simulink model "LGS_allFaultsDeselected"  (R2019b)
settings: Solver=FixedStepDiscrete  StartTime=0.0  StopTime=45.0  FixedStep=0.1  RelTol=1e-3
model workspace (MAT data in the model file):
  fipData : object (value not decoded)
  fipName : object (value not decoded)
  stepSize = 0.1
libraries: LibFaultInjectionControls x190, commrandsrc3 x70, simulink x3, LibFailureCondition x1
(part 7 of 41)

== system LGS_allFaultsDeselected/Digital Part/Computing module2/GenericMonitoring3 ==
  In1 : Inport
  AND : Logic  Inputs=3  IconShape=distinctive  AllPortsSameDT=off  OutDataTypeStr=boolean
  Bus Selector : BusSelector  OutputSignals=signal1,signal2,signal3
  GenericMonitoring2 : Stateflow chart  TreatAsAtomicUnit=on
  Logical Operator1 : Logic  Operator=XOR  AllPortsSameDT=off  OutDataTypeStr=boolean
  Logical Operator2 : Logic  Operator=XOR  AllPortsSameDT=off  OutDataTypeStr=boolean
  Logical Operator3 : Logic  Operator=NOT  AllPortsSameDT=off  OutDataTypeStr=boolean
  Logical Operator4 : Logic  Operator=NOT  AllPortsSameDT=off  OutDataTypeStr=boolean
  Switch : Switch  Criteria=u2 > Threshold
  Switch1 : Switch  Criteria=u2 > Threshold
  Switch2 : Switch  Criteria=u2 > Threshold
  Signal : Outport  OutDataTypeStr=boolean
  Anomaly : Outport  Port=2  OutDataTypeStr=boolean
  wires:
  Bus Selector/1 -> GenericMonitoring2/1(Channel1), Logical Operator1/1, Switch1/1, Switch/1, AND/1  "<signal1>"
  Bus Selector/2 -> AND/2, GenericMonitoring2/2(Channel2), Logical Operator1/2, Logical Operator2/1, Switch2/1  "<signal2>"
  Bus Selector/3 -> AND/3, GenericMonitoring2/3(Channel3), Logical Operator2/2, Switch2/3  "<signal3>"
  In1/1 -> Bus Selector/1
  AND/1 -> Switch/2
  GenericMonitoring2/1(anomaly) -> Anomaly/1
  Switch/1 -> Signal/1
  Logical Operator4/1 -> Switch1/2
  Logical Operator2/1 -> Logical Operator3/1
  Switch2/1 -> Switch1/3
  Switch1/1 -> Switch/3
  Logical Operator3/1 -> Switch2/2
  Logical Operator1/1 -> Logical Operator4/1

== system LGS_allFaultsDeselected/Digital Part/Computing module2/GenericMonitoring4 ==
  In1 : Inport
  AND : Logic  Inputs=3  IconShape=distinctive  AllPortsSameDT=off  OutDataTypeStr=boolean
  Bus Selector : BusSelector  OutputSignals=signal1,signal2,signal3
  GenericMonitoring2 : Stateflow chart  TreatAsAtomicUnit=on
  Logical Operator1 : Logic  Operator=XOR  AllPortsSameDT=off  OutDataTypeStr=boolean
  Logical Operator2 : Logic  Operator=XOR  AllPortsSameDT=off  OutDataTypeStr=boolean
  Logical Operator3 : Logic  Operator=NOT  AllPortsSameDT=off  OutDataTypeStr=boolean
  Logical Operator4 : Logic  Operator=NOT  AllPortsSameDT=off  OutDataTypeStr=boolean
  Switch : Switch  Criteria=u2 > Threshold
  Switch1 : Switch  Criteria=u2 > Threshold
  Switch2 : Switch  Criteria=u2 > Threshold
  Signal : Outport  OutDataTypeStr=boolean
  Anomaly : Outport  Port=2  OutDataTypeStr=boolean
  wires:
  Bus Selector/1 -> GenericMonitoring2/1(Channel1), Logical Operator1/1, Switch1/1, Switch/1, AND/1  "<signal1>"
  Bus Selector/2 -> AND/2, GenericMonitoring2/2(Channel2), Logical Operator1/2, Logical Operator2/1, Switch2/1  "<signal2>"
  Bus Selector/3 -> AND/3, GenericMonitoring2/3(Channel3), Logical Operator2/2, Switch2/3  "<signal3>"
  In1/1 -> Bus Selector/1
  AND/1 -> Switch/2
  GenericMonitoring2/1(anomaly) -> Anomaly/1
  Switch/1 -> Signal/1
  Logical Operator4/1 -> Switch1/2
  Logical Operator2/1 -> Logical Operator3/1
  Switch2/1 -> Switch1/3
  Switch1/1 -> Switch/3
  Logical Operator3/1 -> Switch2/2
  Logical Operator1/1 -> Logical Operator4/1

== system LGS_allFaultsDeselected/Digital Part/Computing module2/GenericMonitoring5 ==
  In1 : Inport
  AND : Logic  Inputs=3  IconShape=distinctive  AllPortsSameDT=off  OutDataTypeStr=boolean
  Bus Selector : BusSelector  OutputSignals=signal1,signal2,signal3
  GenericMonitoring2 : Stateflow chart  TreatAsAtomicUnit=on
  Logical Operator1 : Logic  Operator=XOR  AllPortsSameDT=off  OutDataTypeStr=boolean
  Logical Operator2 : Logic  Operator=XOR  AllPortsSameDT=off  OutDataTypeStr=boolean
  Logical Operator3 : Logic  Operator=NOT  AllPortsSameDT=off  OutDataTypeStr=boolean
  Logical Operator4 : Logic  Operator=NOT  AllPortsSameDT=off  OutDataTypeStr=boolean
  Switch : Switch  Criteria=u2 > Threshold
  Switch1 : Switch  Criteria=u2 > Threshold
  Switch2 : Switch  Criteria=u2 > Threshold
  Signal : Outport  OutDataTypeStr=boolean
  Anomaly : Outport  Port=2  OutDataTypeStr=boolean
  wires:
  Bus Selector/1 -> GenericMonitoring2/1(Channel1), Logical Operator1/1, Switch1/1, Switch/1, AND/1  "<signal1>"
  Bus Selector/2 -> AND/2, GenericMonitoring2/2(Channel2), Logical Operator1/2, Logical Operator2/1, Switch2/1  "<signal2>"
  Bus Selector/3 -> AND/3, GenericMonitoring2/3(Channel3), Logical Operator2/2, Switch2/3  "<signal3>"
  In1/1 -> Bus Selector/1
  AND/1 -> Switch/2
  GenericMonitoring2/1(anomaly) -> Anomaly/1
  Switch/1 -> Signal/1
  Logical Operator4/1 -> Switch1/2
  Logical Operator2/1 -> Logical Operator3/1
  Switch2/1 -> Switch1/3
  Switch1/1 -> Switch/3
  Logical Operator3/1 -> Switch2/2
  Logical Operator1/1 -> Logical Operator4/1

== system LGS_allFaultsDeselected/Digital Part/Computing module2/GenericMonitoring6 ==
  In1 : Inport
  AND : Logic  Inputs=3  IconShape=distinctive  AllPortsSameDT=off  OutDataTypeStr=boolean
  Bus Selector : BusSelector  OutputSignals=signal1,signal2,signal3
  GenericMonitoring2 : Stateflow chart  TreatAsAtomicUnit=on
  Logical Operator1 : Logic  Operator=XOR  AllPortsSameDT=off  OutDataTypeStr=boolean
  Logical Operator2 : Logic  Operator=XOR  AllPortsSameDT=off  OutDataTypeStr=boolean
  Logical Operator3 : Logic  Operator=NOT  AllPortsSameDT=off  OutDataTypeStr=boolean
  Logical Operator4 : Logic  Operator=NOT  AllPortsSameDT=off  OutDataTypeStr=boolean
  Switch : Switch  Criteria=u2 > Threshold
  Switch1 : Switch  Criteria=u2 > Threshold
  Switch2 : Switch  Criteria=u2 > Threshold
  Signal : Outport  OutDataTypeStr=boolean
  Anomaly : Outport  Port=2  OutDataTypeStr=boolean
  wires:
  Bus Selector/1 -> GenericMonitoring2/1(Channel1), Logical Operator1/1, Switch1/1, Switch/1, AND/1  "<signal1>"
  Bus Selector/2 -> AND/2, GenericMonitoring2/2(Channel2), Logical Operator1/2, Logical Operator2/1, Switch2/1  "<signal2>"
  Bus Selector/3 -> AND/3, GenericMonitoring2/3(Channel3), Logical Operator2/2, Switch2/3  "<signal3>"
  In1/1 -> Bus Selector/1
  AND/1 -> Switch/2
  GenericMonitoring2/1(anomaly) -> Anomaly/1
  Switch/1 -> Signal/1
  Logical Operator4/1 -> Switch1/2
  Logical Operator2/1 -> Logical Operator3/1
  Switch2/1 -> Switch1/3
  Switch1/1 -> Switch/3
  Logical Operator3/1 -> Switch2/2
  Logical Operator1/1 -> Logical Operator4/1

== system LGS_allFaultsDeselected/Digital Part/Computing module2/GenericMonitoring7 ==
  In1 : Inport
  AND : Logic  Inputs=3  IconShape=distinctive  AllPortsSameDT=off  OutDataTypeStr=boolean
  Bus Selector : BusSelector  OutputSignals=signal1,signal2,signal3
  GenericMonitoring2 : Stateflow chart  TreatAsAtomicUnit=on
  Logical Operator1 : Logic  Operator=XOR  AllPortsSameDT=off  OutDataTypeStr=boolean
  Logical Operator2 : Logic  Operator=XOR  AllPortsSameDT=off  OutDataTypeStr=boolean
  Logical Operator3 : Logic  Operator=NOT  AllPortsSameDT=off  OutDataTypeStr=boolean
  Logical Operator4 : Logic  Operator=NOT  AllPortsSameDT=off  OutDataTypeStr=boolean
  Switch : Switch  Criteria=u2 > Threshold
  Switch1 : Switch  Criteria=u2 > Threshold
  Switch2 : Switch  Criteria=u2 > Threshold
  Signal : Outport  OutDataTypeStr=boolean
  Anomaly : Outport  Port=2  OutDataTypeStr=boolean
  wires:
  Bus Selector/1 -> GenericMonitoring2/1(Channel1), Logical Operator1/1, Switch1/1, Switch/1, AND/1  "<signal1>"
  Bus Selector/2 -> AND/2, GenericMonitoring2/2(Channel2), Logical Operator1/2, Logical Operator2/1, Switch2/1  "<signal2>"
  Bus Selector/3 -> AND/3, GenericMonitoring2/3(Channel3), Logical Operator2/2, Switch2/3  "<signal3>"
  In1/1 -> Bus Selector/1
  AND/1 -> Switch/2
  GenericMonitoring2/1(anomaly) -> Anomaly/1
  Switch/1 -> Signal/1
  Logical Operator4/1 -> Switch1/2
  Logical Operator2/1 -> Logical Operator3/1
  Switch2/1 -> Switch1/3
  Switch1/1 -> Switch/3
  Logical Operator3/1 -> Switch2/2
  Logical Operator1/1 -> Logical Operator4/1

== system LGS_allFaultsDeselected/Digital Part/Computing module2/GenericMonitoring8 ==
  In1 : Inport
  AND : Logic  Inputs=3  IconShape=distinctive  AllPortsSameDT=off  OutDataTypeStr=boolean
  Bus Selector : BusSelector  OutputSignals=signal1,signal2,signal3
  GenericMonitoring2 : Stateflow chart  TreatAsAtomicUnit=on
  Logical Operator1 : Logic  Operator=XOR  AllPortsSameDT=off  OutDataTypeStr=boolean
  Logical Operator2 : Logic  Operator=XOR  AllPortsSameDT=off  OutDataTypeStr=boolean
  Logical Operator3 : Logic  Operator=NOT  AllPortsSameDT=off  OutDataTypeStr=boolean
  Logical Operator4 : Logic  Operator=NOT  AllPortsSameDT=off  OutDataTypeStr=boolean
  Switch : Switch  Criteria=u2 > Threshold
  Switch1 : Switch  Criteria=u2 > Threshold
  Switch2 : Switch  Criteria=u2 > Threshold
  Signal : Outport  OutDataTypeStr=boolean
  Anomaly : Outport  Port=2  OutDataTypeStr=boolean
  wires:
  Bus Selector/1 -> GenericMonitoring2/1(Channel1), Logical Operator1/1, Switch1/1, Switch/1, AND/1  "<signal1>"
  Bus Selector/2 -> AND/2, GenericMonitoring2/2(Channel2), Logical Operator1/2, Logical Operator2/1, Switch2/1  "<signal2>"
  Bus Selector/3 -> AND/3, GenericMonitoring2/3(Channel3), Logical Operator2/2, Switch2/3  "<signal3>"
  In1/1 -> Bus Selector/1
  AND/1 -> Switch/2
  GenericMonitoring2/1(anomaly) -> Anomaly/1
  Switch/1 -> Signal/1
  Logical Operator4/1 -> Switch1/2
  Logical Operator2/1 -> Logical Operator3/1
  Switch2/1 -> Switch1/3
  Switch1/1 -> Switch/3
  Logical Operator3/1 -> Switch2/2
  Logical Operator1/1 -> Logical Operator4/1

== system LGS_allFaultsDeselected/Digital Part/Computing module2/GenericMonitoring9 ==
  In1 : Inport
  AND : Logic  Inputs=3  IconShape=distinctive  AllPortsSameDT=off  OutDataTypeStr=boolean
  Bus Selector : BusSelector  OutputSignals=signal1,signal2,signal3
  GenericMonitoring2 : Stateflow chart  TreatAsAtomicUnit=on
  Logical Operator1 : Logic  Operator=XOR  AllPortsSameDT=off  OutDataTypeStr=boolean
  Logical Operator2 : Logic  Operator=XOR  AllPortsSameDT=off  OutDataTypeStr=boolean
  Logical Operator3 : Logic  Operator=NOT  AllPortsSameDT=off  OutDataTypeStr=boolean
  Logical Operator4 : Logic  Operator=NOT  AllPortsSameDT=off  OutDataTypeStr=boolean
  Switch : Switch  Criteria=u2 > Threshold
  Switch1 : Switch  Criteria=u2 > Threshold
  Switch2 : Switch  Criteria=u2 > Threshold
  Signal : Outport  OutDataTypeStr=boolean
  Anomaly : Outport  Port=2  OutDataTypeStr=boolean
  wires:
  Bus Selector/1 -> GenericMonitoring2/1(Channel1), Logical Operator1/1, Switch1/1, Switch/1, AND/1  "<signal1>"
  Bus Selector/2 -> AND/2, GenericMonitoring2/2(Channel2), Logical Operator1/2, Logical Operator2/1, Switch2/1  "<signal2>"
  Bus Selector/3 -> AND/3, GenericMonitoring2/3(Channel3), Logical Operator2/2, Switch2/3  "<signal3>"
  In1/1 -> Bus Selector/1
  AND/1 -> Switch/2
  GenericMonitoring2/1(anomaly) -> Anomaly/1
  Switch/1 -> Signal/1
  Logical Operator4/1 -> Switch1/2
  Logical Operator2/1 -> Logical Operator3/1
  Switch2/1 -> Switch1/3
  Switch1/1 -> Switch/3
  Logical Operator3/1 -> Switch2/2
  Logical Operator1/1 -> Logical Operator4/1

== system LGS_allFaultsDeselected/Digital Part/Computing module2/ReactToHandleChange ==
  In1 : Inport  OutDataTypeStr=boolean
  Delay1 : Delay  DelayLength=1  InitialCondition=0
  Delay2 : Delay  DelayLength=1  InitialCondition=0
  Logical Operator : Logic  AllPortsSameDT=off  OutDataTypeStr=boolean
  Logical Operator1 : Logic  Operator=NOT  AllPortsSameDT=off  OutDataTypeStr=boolean
  Logical Operator2 : Logic  AllPortsSameDT=off  OutDataTypeStr=boolean
  Logical Operator3 : Logic  Operator=NOT  AllPortsSameDT=off  OutDataTypeStr=boolean
  Extending : Outport  OutDataTypeStr=boolean
  Retracting : Outport  Port=2  OutDataTypeStr=boolean
  wires:
  In1/1 -> Delay2/1, Logical Operator2/2, Logical Operator1/1, Delay1/1
  Delay1/1 -> Logical Operator/1
  Logical Operator1/1 -> Logical Operator/2
  Logical Operator/1 -> Extending/1
  Logical Operator3/1 -> Logical Operator2/1
  Delay2/1 -> Logical Operator3/1
  Logical Operator2/1 -> Retracting/1

== system LGS_allFaultsDeselected/Doors/EV close doors/EV close doors FIP ==
  In1 : Inport
  Blocked closed : Subsystem  mask(FailureMode){isActive=off, isDSF=off, Value=false, FailureRate=1.0E-3, useDefaultMt_copy=off, MaintenanceTask=0, useDefaultMt=off, RiskTime=0, useDefaultRt=off, File=[], DSFjson=JSON}
      mask prompts: isActive "is Active"; isDSF "DSF Trigger"; Value "Bool Value"; useDefaultMt_copy "set"; useDefaultMt "set"; useDefaultRt "set"
      mask TypeOptions isActive: Trigger FIP/Active
      mask TypeOptions isDSF: Trigger FIP/isDSF
      mask Callback isDSF:
      | a = Simulink.Mask.get(gcb);
      | disp(a);
      | d = a.DialogControls();
      | disp(d);
      | for i = 1:size(d,2)
      |     if strcmp(d(i).Name, 'ParameterGroupVar')
      |         basicFip_ctrl = d(i).getDialogControl('BasicFipParam');
      |         dsFip_ctrl = d(i).getDialogControl('DSFipParam');
      | 
      |         if strcmp(get_param(gcb, 'isDSF'), 'on')
      | %            basicFip_ctrl.Visible = 'off';
      |             basicFip_ctrl.Enabled = 'off';
      | 
      |             dsFip_ctrl.Enabled = 'on';
      | %            dsFip_ctrl.Visible = 'on';
      |         else
      |             basicFip_ctrl.Enabled = 'on';
      | %            basicFip_ctrl.Visible = 'on';
      | 
      | %            dsFip_ctrl.Visible = 'off';
      |             dsFip_ctrl.Enabled = 'off';
      |         end
      |     end
      | end
      mask TypeOptions Value: CommitValue/Value
      mask TypeOptions FailureRate: Trigger FIP/FailureRate
      mask Callback useDefaultMt_copy:
      | a = Simulink.Mask.get(gcb);
      | d = a.Parameters();
      | for i = 1:size(d,2)
      |     if strcmp(d(i).Name, 'MaintenanceTask')
      |         if strcmp(get_param(gcb, 'useDefaultMt'), 'off')
      |             set_param(gcb,'MaintenanceTask', '0')
      |             d(i).Enabled = 'off';
      |         else
      |             d(i).Enabled = 'on';
      |         end
      |     end
      | end
      mask TypeOptions MaintenanceTask: Trigger FIP/MaintenanceTask
      mask Callback useDefaultMt:
      | a = Simulink.Mask.get(gcb);
      | d = a.Parameters();
      | for i = 1:size(d,2)
      |     if strcmp(d(i).Name, 'MaintenanceTask')
      |         if strcmp(get_param(gcb, 'useDefaultMt'), 'off')
      |             set_param(gcb,'MaintenanceTask', '0')
      |             d(i).Enabled = 'off';
      |         else
      |             d(i).Enabled = 'on';
      |         end
      |     end
      | end
      mask TypeOptions RiskTime: Trigger FIP/RiskTime
      mask Callback useDefaultRt:
      | a = Simulink.Mask.get(gcb);
      | d = a.Parameters();
      | for i = 1:size(d,2)
      |     if strcmp(d(i).Name, 'RiskTime')
      |         if strcmp(get_param(gcb, 'useDefaultRt'), 'off')
      |             set_param(gcb,'RiskTime', '0')
      |             d(i).Enabled = 'off';
      |         else
      |             d(i).Enabled = 'on';
      |         end
      |     end
      | end
      mask TypeOptions DSFjson: Trigger FIP/DSFjson
      mask DialogControl DescGroupVar Prompt: Bool
      mask DialogControl DescTextVar Prompt: Controls for a fault with boolean as result type
      mask DialogControl BasicFipBehavior Prompt: Failure Mode Behavior
      mask DialogControl BasicFipParamTab Prompt: Failure Mode Occurrence
      mask DialogControl BasicFipParam Prompt: Parameters
      mask DialogControl FailureRate_label Prompt: Failure Rate [1/h]
      mask DialogControl MaintenanceTask_label Prompt: Maintenance Task [h]
      mask DialogControl RiskTime_label Prompt: Risk time [h]
      mask DialogControl DSFipParamTab Prompt: Dependent System Information
      mask DialogControl DSFipParam Prompt: Parameters
      mask DialogControl LoadCSV Prompt: Browse
      mask DialogControl LoadCSV Callback:
      | [file,path,indx] = uigetfile('*.csv');
      | try
      |     set_param(gcb, 'File', append(path,file));
      |     file = fopen(append(path,file));
      | 
      |     fips = {};
      |     cutsets = {};
      | 
      |     line = fgetl(file);
      |     while ischar(line)
      |         disp(join([' > Processing: ',line]));
      |         splitString = split(line, ';');
      |         if isequal(splitString{1}, 'Cut set')
      |             disp('   > Found Cut set');
      |             cs = splitString(2:end-1);
      |             disp(cs);
      |             cutsets{end+1} = cs';
      |         else
      |             disp('   > Found FIP');
      |             if ~isequal("h", splitString(7))
      |                 disp('no time format except hour is supported');
      |             end
      |             fip = {};
      |             fip.id = splitString(1);
      |             fip.path = splitString(3);
      |             fip.rate = splitString(4);
      |             fip.checkInterval = splitString(6);
      |             disp(fip);
      |             fips{end+1} = fip;
      |         end
      |         line = fgetl(file);
      |     end
      | 
      |     fclose(file);
      | 
      |     DSF = {};
      |     DSF.fips = fips;
      |     DSF.cutsets = cutsets;
      | 
      |     VarCSText = jsonencode(DSF);
      |     set_param(gcb, 'DSFjson', VarCSText);
      | catch
      | end
  Blocked open : Subsystem  mask(FailureMode){isActive=off, isDSF=off, Value=true, FailureRate=1.0E-3, useDefaultMt_copy=off, MaintenanceTask=0, useDefaultMt=off, RiskTime=0, useDefaultRt=off, File=[], DSFjson=JSON}
      mask prompts: isActive "is Active"; isDSF "DSF Trigger"; Value "Bool Value"; useDefaultMt_copy "set"; useDefaultMt "set"; useDefaultRt "set"
      mask TypeOptions isActive: Trigger FIP/Active
      mask TypeOptions isDSF: Trigger FIP/isDSF
      mask Callback isDSF:
      | a = Simulink.Mask.get(gcb);
      | disp(a);
      | d = a.DialogControls();
      | disp(d);
      | for i = 1:size(d,2)
      |     if strcmp(d(i).Name, 'ParameterGroupVar')
      |         basicFip_ctrl = d(i).getDialogControl('BasicFipParam');
      |         dsFip_ctrl = d(i).getDialogControl('DSFipParam');
      | 
      |         if strcmp(get_param(gcb, 'isDSF'), 'on')
      | %            basicFip_ctrl.Visible = 'off';
      |             basicFip_ctrl.Enabled = 'off';
      | 
      |             dsFip_ctrl.Enabled = 'on';
      | %            dsFip_ctrl.Visible = 'on';
      |         else
      |             basicFip_ctrl.Enabled = 'on';
      | %            basicFip_ctrl.Visible = 'on';
      | 
      | %            dsFip_ctrl.Visible = 'off';
      |             dsFip_ctrl.Enabled = 'off';
      |         end
      |     end
      | end
      mask TypeOptions Value: CommitValue/Value
      mask TypeOptions FailureRate: Trigger FIP/FailureRate
      mask Callback useDefaultMt_copy:
      | a = Simulink.Mask.get(gcb);
      | d = a.Parameters();
      | for i = 1:size(d,2)
      |     if strcmp(d(i).Name, 'MaintenanceTask')
      |         if strcmp(get_param(gcb, 'useDefaultMt'), 'off')
      |             set_param(gcb,'MaintenanceTask', '0')
      |             d(i).Enabled = 'off';
      |         else
      |             d(i).Enabled = 'on';
      |         end
      |     end
      | end
      mask TypeOptions MaintenanceTask: Trigger FIP/MaintenanceTask
      mask Callback useDefaultMt:
      | a = Simulink.Mask.get(gcb);
      | d = a.Parameters();
      | for i = 1:size(d,2)
      |     if strcmp(d(i).Name, 'MaintenanceTask')
      |         if strcmp(get_param(gcb, 'useDefaultMt'), 'off')
      |             set_param(gcb,'MaintenanceTask', '0')
      |             d(i).Enabled = 'off';
      |         else
      |             d(i).Enabled = 'on';
      |         end
      |     end
      | end
      mask TypeOptions RiskTime: Trigger FIP/RiskTime
      mask Callback useDefaultRt:
      | a = Simulink.Mask.get(gcb);
      | d = a.Parameters();
      | for i = 1:size(d,2)
      |     if strcmp(d(i).Name, 'RiskTime')
      |         if strcmp(get_param(gcb, 'useDefaultRt'), 'off')
      |             set_param(gcb,'RiskTime', '0')
      |             d(i).Enabled = 'off';
      |         else
      |             d(i).Enabled = 'on';
      |         end
      |     end
      | end
      mask TypeOptions DSFjson: Trigger FIP/DSFjson
      mask DialogControl DescGroupVar Prompt: Bool
      mask DialogControl DescTextVar Prompt: Controls for a fault with boolean as result type
      mask DialogControl BasicFipBehavior Prompt: Failure Mode Behavior
      mask DialogControl BasicFipParamTab Prompt: Failure Mode Occurrence
      mask DialogControl BasicFipParam Prompt: Parameters
      mask DialogControl FailureRate_label Prompt: Failure Rate [1/h]
      mask DialogControl MaintenanceTask_label Prompt: Maintenance Task [h]
      mask DialogControl RiskTime_label Prompt: Risk time [h]
      mask DialogControl DSFipParamTab Prompt: Dependent System Information
      mask DialogControl DSFipParam Prompt: Parameters
      mask DialogControl LoadCSV Prompt: Browse
      mask DialogControl LoadCSV Callback:
      | [file,path,indx] = uigetfile('*.csv');
      | try
      |     set_param(gcb, 'File', append(path,file));
      |     file = fopen(append(path,file));
      | 
      |     fips = {};
      |     cutsets = {};
      | 
      |     line = fgetl(file);
      |     while ischar(line)
      |         disp(join([' > Processing: ',line]));
      |         splitString = split(line, ';');
      |         if isequal(splitString{1}, 'Cut set')
      |             disp('   > Found Cut set');
      |             cs = splitString(2:end-1);
      |             disp(cs);
      |             cutsets{end+1} = cs';
      |         else
      |             disp('   > Found FIP');
      |             if ~isequal("h", splitString(7))
      |                 disp('no time format except hour is supported');
      |             end
      |             fip = {};
      |             fip.id = splitString(1);
      |             fip.path = splitString(3);
      |             fip.rate = splitString(4);
      |             fip.checkInterval = splitString(6);
      |             disp(fip);
      |             fips{end+1} = fip;
      |         end
      |         line = fgetl(file);
      |     end
      | 
      |     fclose(file);
      | 
      |     DSF = {};
      |     DSF.fips = fips;
      |     DSF.cutsets = cutsets;
      | 
      |     VarCSText = jsonencode(DSF);
      |     set_param(gcb, 'DSFjson', VarCSText);
      | catch
      | end
  Out1 : Outport
  wires:
  Blocked open/1(Out1) -> Out1/1
  Blocked closed/1(Out1) -> Blocked open/1(In1)
  In1/1 -> Blocked closed/1(In1)

== system LGS_allFaultsDeselected/Doors/EV open doors/EV open doors FIP ==
  In1 : Inport
  Blocked closed : Subsystem  mask(FailureMode){isActive=off, isDSF=off, Value=false, FailureRate=1.0E-3, useDefaultMt_copy=off, MaintenanceTask=0, useDefaultMt=off, RiskTime=0, useDefaultRt=off, File=[], DSFjson=JSON}
      mask prompts: isActive "is Active"; isDSF "DSF Trigger"; Value "Bool Value"; useDefaultMt_copy "set"; useDefaultMt "set"; useDefaultRt "set"
      mask TypeOptions isActive: Trigger FIP/Active
      mask TypeOptions isDSF: Trigger FIP/isDSF
      mask Callback isDSF:
      | a = Simulink.Mask.get(gcb);
      | disp(a);
      | d = a.DialogControls();
      | disp(d);
      | for i = 1:size(d,2)
      |     if strcmp(d(i).Name, 'ParameterGroupVar')
      |         basicFip_ctrl = d(i).getDialogControl('BasicFipParam');
      |         dsFip_ctrl = d(i).getDialogControl('DSFipParam');
      | 
      |         if strcmp(get_param(gcb, 'isDSF'), 'on')
      | %            basicFip_ctrl.Visible = 'off';
      |             basicFip_ctrl.Enabled = 'off';
      | 
      |             dsFip_ctrl.Enabled = 'on';
      | %            dsFip_ctrl.Visible = 'on';
      |         else
      |             basicFip_ctrl.Enabled = 'on';
      | %            basicFip_ctrl.Visible = 'on';
      | 
      | %            dsFip_ctrl.Visible = 'off';
      |             dsFip_ctrl.Enabled = 'off';
      |         end
      |     end
      | end
      mask TypeOptions Value: CommitValue/Value
      mask TypeOptions FailureRate: Trigger FIP/FailureRate
      mask Callback useDefaultMt_copy:
      | a = Simulink.Mask.get(gcb);
      | d = a.Parameters();
      | for i = 1:size(d,2)
      |     if strcmp(d(i).Name, 'MaintenanceTask')
      |         if strcmp(get_param(gcb, 'useDefaultMt'), 'off')
      |             set_param(gcb,'MaintenanceTask', '0')
      |             d(i).Enabled = 'off';
      |         else
      |             d(i).Enabled = 'on';
      |         end
      |     end
      | end
      mask TypeOptions MaintenanceTask: Trigger FIP/MaintenanceTask
      mask Callback useDefaultMt:
      | a = Simulink.Mask.get(gcb);
      | d = a.Parameters();
      | for i = 1:size(d,2)
      |     if strcmp(d(i).Name, 'MaintenanceTask')
      |         if strcmp(get_param(gcb, 'useDefaultMt'), 'off')
      |             set_param(gcb,'MaintenanceTask', '0')
      |             d(i).Enabled = 'off';
      |         else
      |             d(i).Enabled = 'on';
      |         end
      |     end
      | end
      mask TypeOptions RiskTime: Trigger FIP/RiskTime
      mask Callback useDefaultRt:
      | a = Simulink.Mask.get(gcb);
      | d = a.Parameters();
      | for i = 1:size(d,2)
      |     if strcmp(d(i).Name, 'RiskTime')
      |         if strcmp(get_param(gcb, 'useDefaultRt'), 'off')
      |             set_param(gcb,'RiskTime', '0')
      |             d(i).Enabled = 'off';
      |         else
      |             d(i).Enabled = 'on';
      |         end
      |     end
      | end
      mask TypeOptions DSFjson: Trigger FIP/DSFjson
      mask DialogControl DescGroupVar Prompt: Bool
      mask DialogControl DescTextVar Prompt: Controls for a fault with boolean as result type
      mask DialogControl BasicFipBehavior Prompt: Failure Mode Behavior
      mask DialogControl BasicFipParamTab Prompt: Failure Mode Occurrence
      mask DialogControl BasicFipParam Prompt: Parameters
      mask DialogControl FailureRate_label Prompt: Failure Rate [1/h]
      mask DialogControl MaintenanceTask_label Prompt: Maintenance Task [h]
      mask DialogControl RiskTime_label Prompt: Risk time [h]
      mask DialogControl DSFipParamTab Prompt: Dependent System Information
      mask DialogControl DSFipParam Prompt: Parameters
      mask DialogControl LoadCSV Prompt: Browse
      mask DialogControl LoadCSV Callback:
      | [file,path,indx] = uigetfile('*.csv');
      | try
      |     set_param(gcb, 'File', append(path,file));
      |     file = fopen(append(path,file));
      | 
      |     fips = {};
      |     cutsets = {};
      | 
      |     line = fgetl(file);
      |     while ischar(line)
      |         disp(join([' > Processing: ',line]));
      |         splitString = split(line, ';');
      |         if isequal(splitString{1}, 'Cut set')
      |             disp('   > Found Cut set');
      |             cs = splitString(2:end-1);
      |             disp(cs);
      |             cutsets{end+1} = cs';
      |         else
      |             disp('   > Found FIP');
      |             if ~isequal("h", splitString(7))
      |                 disp('no time format except hour is supported');
      |             end
      |             fip = {};
      |             fip.id = splitString(1);
      |             fip.path = splitString(3);
      |             fip.rate = splitString(4);
      |             fip.checkInterval = splitString(6);
      |             disp(fip);
      |             fips{end+1} = fip;
      |         end
      |         line = fgetl(file);
      |     end
      | 
      |     fclose(file);
      | 
      |     DSF = {};
      |     DSF.fips = fips;
      |     DSF.cutsets = cutsets;
      | 
      |     VarCSText = jsonencode(DSF);
      |     set_param(gcb, 'DSFjson', VarCSText);
      | catch
      | end
  Blocked open : Subsystem  mask(FailureMode){isActive=off, isDSF=off, Value=true, FailureRate=1.0E-3, useDefaultMt_copy=off, MaintenanceTask=0, useDefaultMt=off, RiskTime=0, useDefaultRt=off, File=[], DSFjson=JSON}
      mask prompts: isActive "is Active"; isDSF "DSF Trigger"; Value "Bool Value"; useDefaultMt_copy "set"; useDefaultMt "set"; useDefaultRt "set"
      mask TypeOptions isActive: Trigger FIP/Active
      mask TypeOptions isDSF: Trigger FIP/isDSF
      mask Callback isDSF:
      | a = Simulink.Mask.get(gcb);
      | disp(a);
      | d = a.DialogControls();
      | disp(d);
      | for i = 1:size(d,2)
      |     if strcmp(d(i).Name, 'ParameterGroupVar')
      |         basicFip_ctrl = d(i).getDialogControl('BasicFipParam');
      |         dsFip_ctrl = d(i).getDialogControl('DSFipParam');
      | 
      |         if strcmp(get_param(gcb, 'isDSF'), 'on')
      | %            basicFip_ctrl.Visible = 'off';
      |             basicFip_ctrl.Enabled = 'off';
      | 
      |             dsFip_ctrl.Enabled = 'on';
      | %            dsFip_ctrl.Visible = 'on';
      |         else
      |             basicFip_ctrl.Enabled = 'on';
      | %            basicFip_ctrl.Visible = 'on';
      | 
      | %            dsFip_ctrl.Visible = 'off';
      |             dsFip_ctrl.Enabled = 'off';
      |         end
      |     end
      | end
      mask TypeOptions Value: CommitValue/Value
      mask TypeOptions FailureRate: Trigger FIP/FailureRate
      mask Callback useDefaultMt_copy:
      | a = Simulink.Mask.get(gcb);
      | d = a.Parameters();
      | for i = 1:size(d,2)
      |     if strcmp(d(i).Name, 'MaintenanceTask')
      |         if strcmp(get_param(gcb, 'useDefaultMt'), 'off')
      |             set_param(gcb,'MaintenanceTask', '0')
      |             d(i).Enabled = 'off';
      |         else
      |             d(i).Enabled = 'on';
      |         end
      |     end
      | end
      mask TypeOptions MaintenanceTask: Trigger FIP/MaintenanceTask
      mask Callback useDefaultMt:
      | a = Simulink.Mask.get(gcb);
      | d = a.Parameters();
      | for i = 1:size(d,2)
      |     if strcmp(d(i).Name, 'MaintenanceTask')
      |         if strcmp(get_param(gcb, 'useDefaultMt'), 'off')
      |             set_param(gcb,'MaintenanceTask', '0')
      |             d(i).Enabled = 'off';
      |         else
      |             d(i).Enabled = 'on';
      |         end
      |     end
      | end
      mask TypeOptions RiskTime: Trigger FIP/RiskTime
      mask Callback useDefaultRt:
      | a = Simulink.Mask.get(gcb);
      | d = a.Parameters();
      | for i = 1:size(d,2)
      |     if strcmp(d(i).Name, 'RiskTime')
      |         if strcmp(get_param(gcb, 'useDefaultRt'), 'off')
      |             set_param(gcb,'RiskTime', '0')
      |             d(i).Enabled = 'off';
      |         else
      |             d(i).Enabled = 'on';
      |         end
      |     end
      | end
      mask TypeOptions DSFjson: Trigger FIP/DSFjson
      mask DialogControl DescGroupVar Prompt: Bool
      mask DialogControl DescTextVar Prompt: Controls for a fault with boolean as result type
      mask DialogControl BasicFipBehavior Prompt: Failure Mode Behavior
      mask DialogControl BasicFipParamTab Prompt: Failure Mode Occurrence
      mask DialogControl BasicFipParam Prompt: Parameters
      mask DialogControl FailureRate_label Prompt: Failure Rate [1/h]
      mask DialogControl MaintenanceTask_label Prompt: Maintenance Task [h]
      mask DialogControl RiskTime_label Prompt: Risk time [h]
      mask DialogControl DSFipParamTab Prompt: Dependent System Information
      mask DialogControl DSFipParam Prompt: Parameters
      mask DialogControl LoadCSV Prompt: Browse
      mask DialogControl LoadCSV Callback:
      | [file,path,indx] = uigetfile('*.csv');
      | try
      |     set_param(gcb, 'File', append(path,file));
      |     file = fopen(append(path,file));
      | 
      |     fips = {};
      |     cutsets = {};
      | 
      |     line = fgetl(file);
      |     while ischar(line)
      |         disp(join([' > Processing: ',line]));
      |         splitString = split(line, ';');
      |         if isequal(splitString{1}, 'Cut set')
      |             disp('   > Found Cut set');
      |             cs = splitString(2:end-1);
      |             disp(cs);
      |             cutsets{end+1} = cs';
      |         else
      |             disp('   > Found FIP');
      |             if ~isequal("h", splitString(7))
      |                 disp('no time format except hour is supported');
      |             end
      |             fip = {};
      |             fip.id = splitString(1);
      |             fip.path = splitString(3);
      |             fip.rate = splitString(4);
      |             fip.checkInterval = splitString(6);
      |             disp(fip);
      |             fips{end+1} = fip;
      |         end
      |         line = fgetl(file);
      |     end
      | 
      |     fclose(file);
      | 
      |     DSF = {};
      |     DSF.fips = fips;
      |     DSF.cutsets = cutsets;
      | 
      |     VarCSText = jsonencode(DSF);
      |     set_param(gcb, 'DSFjson', VarCSText);
      | catch
      | end
  Out1 : Outport
  wires:
  Blocked open/1(Out1) -> Out1/1
  Blocked closed/1(Out1) -> Blocked open/1(In1)
  In1/1 -> Blocked closed/1(In1)

== system LGS_allFaultsDeselected/Doors/front door zylinder/sensor locked closed ==
  note: [true, false]
  note: [true, false]
  note: [true, false]
  sensor input : Inport  OutDataTypeStr=boolean
  Bus Creator3 : BusCreator  Inputs=3
  FIP1 : Subsystem
  FIP2 : Subsystem
  FIP3 : Subsystem
  sensor output : Outport
  wires:
  FIP2/1(Out1) -> Bus Creator3/2  "signal2"
  FIP1/1(Out1) -> Bus Creator3/1  "signal1"
  FIP3/1(Out1) -> Bus Creator3/3  "signal3"
  sensor input/1 -> FIP2/1(In1), FIP1/1(In1), FIP3/1(In1)
  Bus Creator3/1 -> sensor output/1

== system LGS_allFaultsDeselected/Doors/front door zylinder/sensor open ==
  note: [true, false]
  note: [true, false]
  note: [true, false]
  sensor input : Inport  OutDataTypeStr=boolean
  Bus Creator3 : BusCreator  Inputs=3
  FIP1 : Subsystem
  FIP2 : Subsystem
  FIP3 : Subsystem
  sensor output : Outport
  wires:
  FIP2/1(Out1) -> Bus Creator3/2  "signal2"
  FIP1/1(Out1) -> Bus Creator3/1  "signal1"
  FIP3/1(Out1) -> Bus Creator3/3  "signal3"
  sensor input/1 -> FIP3/1(In1), FIP2/1(In1), FIP1/1(In1)
  Bus Creator3/1 -> sensor output/1

== system LGS_allFaultsDeselected/Doors/left door zylinder/sensor locked closed ==
  note: [true, false]
  note: [true, false]
  note: [true, false]
  sensor input : Inport  OutDataTypeStr=boolean
  Bus Creator3 : BusCreator  Inputs=3
  FIP1 : Subsystem
  FIP2 : Subsystem
  FIP3 : Subsystem
  sensor output : Outport
  wires:
  FIP2/1(Out1) -> Bus Creator3/2  "signal2"
  FIP1/1(Out1) -> Bus Creator3/1  "signal1"
  FIP3/1(Out1) -> Bus Creator3/3  "signal3"
  sensor input/1 -> FIP3/1(In1), FIP2/1(In1), FIP1/1(In1)
  Bus Creator3/1 -> sensor output/1

== system LGS_allFaultsDeselected/Doors/left door zylinder/sensor open ==
  note: [true, false]
  note: [true, false]
  note: [true, false]
  sensor input : Inport  OutDataTypeStr=boolean
  Bus Creator3 : BusCreator  Inputs=3
  FIP1 : Subsystem
  FIP2 : Subsystem
  FIP3 : Subsystem
  sensor output : Outport
  wires:
  FIP2/1(Out1) -> Bus Creator3/2  "signal2"
  FIP1/1(Out1) -> Bus Creator3/1  "signal1"
  FIP3/1(Out1) -> Bus Creator3/3  "signal3"
  sensor input/1 -> FIP3/1(In1), FIP2/1(In1), FIP1/1(In1)
  Bus Creator3/1 -> sensor output/1

== system LGS_allFaultsDeselected/Doors/right door zylinder/sensor locked closed ==
  note: [true, false]
  note: [true, false]
  note: [true, false]
  sensor input : Inport  OutDataTypeStr=boolean
  Bus Creator3 : BusCreator  Inputs=3
  FIP1 : Subsystem
  FIP2 : Subsystem
  FIP3 : Subsystem
  sensor output : Outport
  wires:
  FIP2/1(Out1) -> Bus Creator3/2  "signal2"
  FIP1/1(Out1) -> Bus Creator3/1  "signal1"
  FIP3/1(Out1) -> Bus Creator3/3  "signal3"
  sensor input/1 -> FIP3/1(In1), FIP2/1(In1), FIP1/1(In1)
  Bus Creator3/1 -> sensor output/1

== system LGS_allFaultsDeselected/Doors/right door zylinder/sensor open ==
  note: [true, false]
  note: [true, false]
  note: [true, false]
  sensor input : Inport  OutDataTypeStr=boolean
  Bus Creator3 : BusCreator  Inputs=3
  FIP1 : Subsystem
  FIP2 : Subsystem
  FIP3 : Subsystem
  sensor output : Outport
  wires:
  FIP2/1(Out1) -> Bus Creator3/2  "signal2"
  FIP1/1(Out1) -> Bus Creator3/1  "signal1"
  FIP3/1(Out1) -> Bus Creator3/3  "signal3"
  sensor input/1 -> FIP2/1(In1), FIP1/1(In1), FIP3/1(In1)
  Bus Creator3/1 -> sensor output/1

== system LGS_allFaultsDeselected/FailureConditionObserver/FC1/ActualSystemCondition ==
  note: This section validates whether the failure condition to be observed will be evaluated. If the
      | last condition evaluates to false, the following conditions will not be evaluated!
      |
      | The last output should be evaluated to a boolean.
  Constant : Constant  Value=true  OutDataTypeStr=boolean
  "Activate Observer " : Outport
  wires:
  Constant/1 -> "Activate Observer "/1

== system LGS_allFaultsDeselected/FailureConditionObserver/FC1/FC_FC1_output ==
  note: Do not change this area!
  note: Here you can model the actual failure condition. The "Actual System Value Dummy" is a value from the current system and the "Nominal Value Dummy"
      | represents a reference value for the failure condition. You can add as much Nominal Values and Acutal System Values as required. Please Remove the
      | Dummy names before flight.
  ActivateObserver : Inport
  Retraction Valve : Inport  Port=2
  Extension Valve : Inport  Port=3
  Logical Operator : Logic  Operator=OR  AllPortsSameDT=off  OutDataTypeStr=boolean
  Logical Operator1 : Logic  Operator=NOT  AllPortsSameDT=off  OutDataTypeStr=boolean
  Logical Operator3 : Logic  AllPortsSameDT=off  OutDataTypeStr=boolean
  ConditionState : Outport
  wires:
  Logical Operator3/1 -> Logical Operator/2
  Logical Operator1/1 -> Logical Operator/1
  Logical Operator/1 -> ConditionState/1
  ActivateObserver/1 -> Logical Operator1/1
  Extension Valve/1 -> Logical Operator3/2
  Retraction Valve/1 -> Logical Operator3/1

== system LGS_allFaultsDeselected/FailureConditionObserver/FC2/ActualSystemCondition ==
  note: This section validates whether the failure condition to be observed will be evaluated. If the
      | last condition evaluates to false, the following conditions will not be evaluated!
      |
      | The last output should be evaluated to a boolean.
  Constant : Constant  Value=true  OutDataTypeStr=boolean
  "Activate Observer " : Outport
  wires:
  Constant/1 -> "Activate Observer "/1

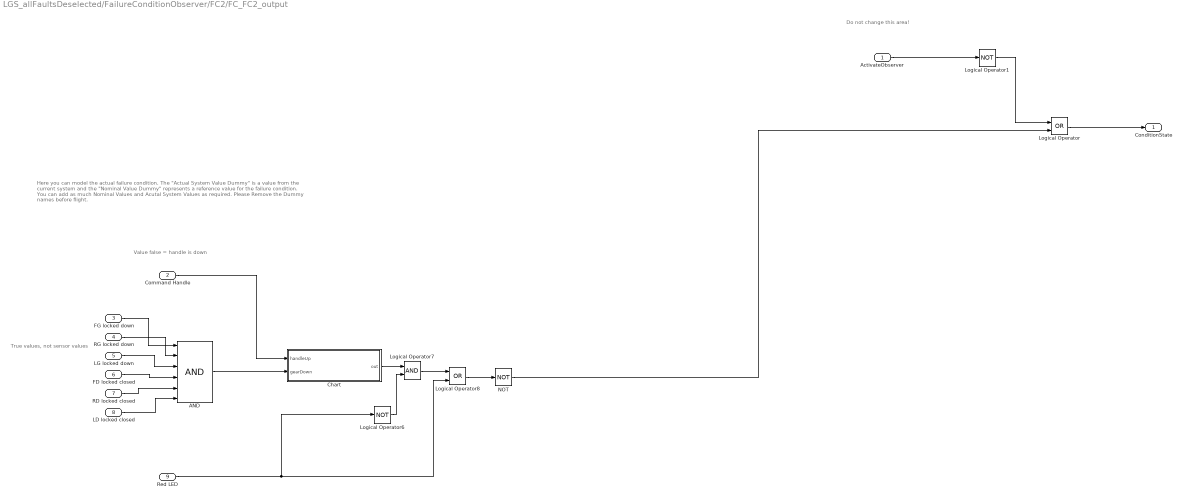
== system LGS_allFaultsDeselected/FailureConditionObserver/FC2/FC_FC2_output ==
  note: Here you can model the actual failure condition. The "Actual System Value Dummy" is a value from the current system and the "Nominal Value Dummy"
      | represents a reference value for the failure condition. You can add as much Nominal Values and Acutal System Values as required. Please Remove the
      | Dummy names before flight.
  note: Do not change this area!
  note: True values, not sensor values
  note: Value false = handle is down
  ActivateObserver : Inport
  Command Handle : Inport  Port=2
  FG locked down : Inport  Port=3
  RG locked down : Inport  Port=4
  LG locked down : Inport  Port=5
  FD locked closed : Inport  Port=6
  RD locked closed : Inport  Port=7
  LD locked closed : Inport  Port=8
  Red LED : Inport  Port=9
  AND : Logic  Inputs=6  IconShape=distinctive  AllPortsSameDT=off  OutDataTypeStr=boolean
  Chart : Stateflow chart  TreatAsAtomicUnit=on
  Logical Operator : Logic  Operator=OR  AllPortsSameDT=off  OutDataTypeStr=boolean
  Logical Operator1 : Logic  Operator=NOT  AllPortsSameDT=off  OutDataTypeStr=boolean
  Logical Operator6 : Logic  Operator=NOT  AllPortsSameDT=off  OutDataTypeStr=boolean
  Logical Operator7 : Logic  AllPortsSameDT=off  OutDataTypeStr=boolean
  Logical Operator8 : Logic  Operator=OR  AllPortsSameDT=off  OutDataTypeStr=boolean
  NOT : Logic  Operator=NOT  AllPortsSameDT=off  OutDataTypeStr=boolean
  ConditionState : Outport
  wires:
  ActivateObserver/1 -> Logical Operator1/1
  Logical Operator/1 -> ConditionState/1
  Logical Operator1/1 -> Logical Operator/1
  Logical Operator8/1 -> NOT/1
  Logical Operator7/1 -> Logical Operator8/1
  Logical Operator6/1 -> Logical Operator7/2
  Red LED/1 -> Logical Operator8/2, Logical Operator6/1
  LG locked down/1 -> AND/3
  RD locked closed/1 -> AND/5
  LD locked closed/1 -> AND/6
  FG locked down/1 -> AND/1
  Command Handle/1 -> Chart/1(handleUp)
  Chart/1(out) -> Logical Operator7/1
  RG locked down/1 -> AND/2
  FD locked closed/1 -> AND/4
  AND/1 -> Chart/2(gearDown)
  NOT/1 -> Logical Operator/2

== system LGS_allFaultsDeselected/FailureConditionObserver/FC3/ActualSystemCondition ==
  note: This section validates whether the failure condition to be observed will be evaluated. If the
      | last condition evaluates to false, the following conditions will not be evaluated!
      |
      | The last output should be evaluated to a boolean.
  Green LED : Inport
  Orange LED : Inport  Port=2
  Red LED : Inport  Port=3
  AND : Logic  Inputs=3  AllPortsSameDT=off  OutDataTypeStr=boolean
  NOT : Logic  Operator=NOT  AllPortsSameDT=off  OutDataTypeStr=boolean
  NOT1 : Logic  Operator=NOT  AllPortsSameDT=off  OutDataTypeStr=boolean
  "Activate Observer " : Outport
  wires:
  AND/1 -> "Activate Observer "/1
  NOT/1 -> AND/2
  Red LED/1 -> NOT1/1
  Orange LED/1 -> NOT/1
  Green LED/1 -> AND/1
  NOT1/1 -> AND/3

== system LGS_allFaultsDeselected/FailureConditionObserver/FC3/FC_FC3_output ==
  note: Here you can model the actual failure condition. The "Actual System Value Dummy" is a value from the current system and the "Nominal Value Dummy"
      | represents a reference value for the failure condition. You can add as much Nominal Values and Acutal System Values as required. Please Remove the
      | Dummy names before flight.
  note: Do not change this area!
  note: True values, not sensor values
  ActivateObserver : Inport
  FG locked down : Inport  Port=2
  RG locked down : Inport  Port=3
  LG locked down : Inport  Port=4
  FD locked closed1 : Inport  Port=5
  RD locked closed1 : Inport  Port=6
  LD locked closed1 : Inport  Port=7
  Logical Operator : Logic  AllPortsSameDT=off  OutDataTypeStr=boolean
  NAND : Logic  Operator=NAND  Inputs=6  IconShape=distinctive  AllPortsSameDT=off  OutDataTypeStr=boolean
  ConditionState : Outport
  wires:
  Logical Operator/1 -> ConditionState/1
  ActivateObserver/1 -> Logical Operator/1
  NAND/1 -> Logical Operator/2
  FG locked down/1 -> NAND/1
  FD locked closed1/1 -> NAND/4
  RD locked closed1/1 -> NAND/5
  RG locked down/1 -> NAND/2
  LG locked down/1 -> NAND/3
  LD locked closed1/1 -> NAND/6
